simulink model "vf_ctrl"  (R2022a)
settings: Solver=FixedStepDiscrete  StartTime=0.0  StopTime=3  FixedStep=T_HF_TASK  RelTol=1e-3  EnableMultiTasking=on
PostLoadFcn:
  | run('init.m')
values from neighbouring files (symbols this model uses):
  INT16_MAX = 32767.0    [vf_ctrl_dd.sldd]
  INT16_MIN = -32768.0    [vf_ctrl_dd.sldd]
  MOTOR_F = 6.3E-6    [vf_ctrl_dd.sldd]
  MOTOR_J = 7.5E-6    [vf_ctrl_dd.sldd]
  MOTOR_PN = 2    [vf_ctrl_dd.sldd]
  MOTOR_PNF = 2.0    [vf_ctrl_dd.sldd]
  MOTOR_TL = 0.001    [vf_ctrl_dd.sldd]
  MOTOR_TYPE = 11.0    [vf_ctrl_dd.sldd]
  PWM_PERIOD_CYCLES = 7200.0    [vf_ctrl_dd.sldd]
  T_HF_TASK = 0.0001    [vf_ctrl_dd.sldd]
  VBUS = 24.0    [vf_ctrl_dd.sldd]
undefined symbols (not defined in the file or in its folder): DiscIntNeverNeededParam
libraries: mcbplantlib x1, autolibpmsmexterior x1
settings Model: DataDictionary=vf_ctrl_dd.sldd  Creator=lww186  LastModifiedBy=YJRQZ777
settings SolverCC: AutoInsertRateTranBlk=on
settings OptimizationCC: DefaultParameterBehavior=Inlined  EnhancedBackFolding=on  PassReuseOutputArgsAs=Individual arguments  ZeroExternalMemoryAtStartup=off  ZeroInternalMemoryAtStartup=off  OptimizeBlockOrder=speed  DifferentSizesBufferReuse=on  OptimizationCustomize=off  EfficientTunableParamExpr=on
settings DebuggingCC: ParameterTunabilityLossMsg=error  UnconnectedInputMsg=warning  UnconnectedOutputMsg=warning  UnconnectedLineMsg=warning
settings HardwareCC: ProdBitPerPointer=32  ProdBitPerSizeT=32  ProdBitPerPtrDiffT=32  ProdLargestAtomicInteger=Long  ProdLargestAtomicFloat=Double  ProdWordSize=32  ProdHWDeviceType=ARM Compatible->ARM Cortex-M
settings SFSimCC: MATLABDynamicMemAlloc=off
settings RTWCC: SystemTargetFile=ert.tlc  GenCodeOnly=on  TemplateMakefile=ert_default_tmf  GenerateReport=on  LaunchReport=on  DLArmComputeVersion=19.05
settings CodeAppCC: ForceParamTrailComments=on  IgnoreCustomStorageClasses=off  OperatorAnnotations=on  SimulinkDataObjDesc=on  SFDataObjDesc=on  InsertBlockDesc=on
settings ERTTargetCC: TargetLangStandard=C99 (ISO)  InlinedParameterPlacement=NonHierarchical  ERTCustomFileTemplate=example_file_process.tlc

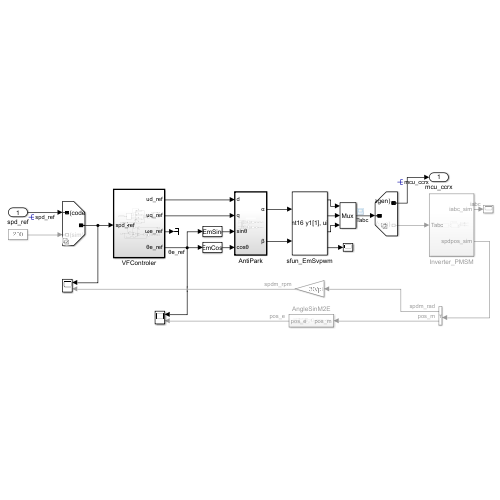
[thumbnail: Simulink's stored preview of the top-level diagram]
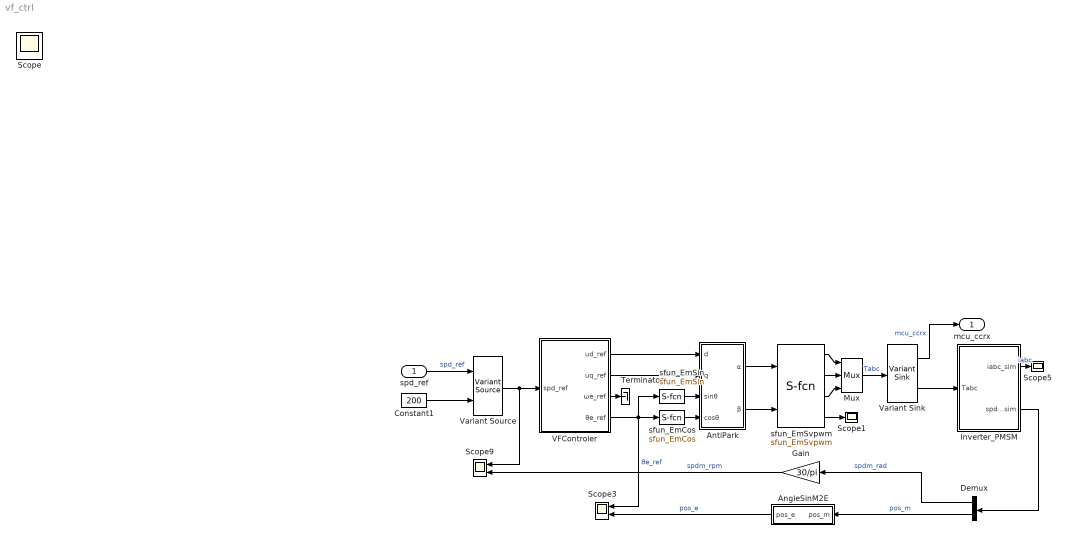
== system vf_ctrl ==
  spd_ref : Inport  OutDataTypeStr=int16
  AngleSinM2E : Subsystem
  AntiPark : Subsystem  TreatAsAtomicUnit=on
      settings: RTWFcnNameOpts=Use subsystem name  RTWFileNameOpts=Use subsystem name
  Constant1 : Constant  Value=200  OutDataTypeStr=int16
  Demux : Demux  Outputs=2
      settings: DisplayOption=none
  Gain : Gain  Gain=30/pi
  Inverter_PMSM : Subsystem
  Mux : Mux  Inputs=3
  Scope1 : Scope
  Scope3 : Scope  NumInputPorts=2
  Scope5 : Scope
  Scope9 : Scope  NumInputPorts=2
  Terminator : Terminator
  VFControler : Subsystem  TreatAsAtomicUnit=on  RTWFcnName=Vfcontroler  RTWFileName=Vfcontroler
      settings: RTWFcnNameOpts=Use subsystem name  RTWFileNameOpts=Use subsystem name
  Variant Sink : VariantSink  VariantControlMode=sim codegen switching  ShowConditionOnBlock=on
  Variant Source : VariantSource  VariantControlMode=sim codegen switching  ShowConditionOnBlock=on
  sfun_EmCos : S-Function  FunctionName=sfun_EmCos  SFunctionDeploymentMode=off  EnableBusSupport=off  mask(Legacy Function){SFunctionSpec=int16 y1 = EmCos( int16 u1 ), ShowSpec=on}
      mask prompts: ShowSpec "显示函数设定"
      mask help:
      | 此模块允许您调用由以下代码继承工具定义指定的已有函数:
      | def.SFunctionName = 'sfun_EmCos';
      | def.OutputFcnSpec = 'int16 y1 = EmCos( int16 u1 )';
      | def.HeaderFiles = {'em_sincos.h'};
      | def.SourceFiles = {'em_sincos.c'};
      | def.IncPaths = {'.\c_code'};
      mask Help: <p>此模块是由代码继承工具自动生成的。有关此工具的详细帮助，请调用<a href="matlab:legacy_code('help')"> legacy_code('help')</a>.</p>
      mask Callback ShowSpec:
      | if strcmp(get_param(gcbh, 'ShowSpec'), 'on')
      |   set_param(gcbh, 'MaskDisplay', sprintf('fprintf(''%s'');', get_param(gcbh, 'SFunctionSpec')));
      | else
      |   set_param(gcbh, 'MaskDisplay', sprintf('fprintf(''%s'');', get_param(gcbh, 'FunctionName')));
      | end
      mask Display: fprintf('int16 y1 = EmCos( int16 u1 )');
  sfun_EmSin : S-Function  FunctionName=sfun_EmSin  SFunctionDeploymentMode=off  EnableBusSupport=off  mask(Legacy Function){SFunctionSpec=int16 y1 = EmSin( int16 u1 ), ShowSpec=on}
      mask prompts: ShowSpec "显示函数设定"
      mask help:
      | 此模块允许您调用由以下代码继承工具定义指定的已有函数:
      | def.SFunctionName = 'sfun_EmSin';
      | def.OutputFcnSpec = 'int16 y1 = EmSin( int16 u1 )';
      | def.HeaderFiles = {'em_sincos.h'};
      | def.SourceFiles = {'em_sincos.c'};
      | def.IncPaths = {'.\c_code'};
      mask Help: <p>此模块是由代码继承工具自动生成的。有关此工具的详细帮助，请调用<a href="matlab:legacy_code('help')"> legacy_code('help')</a>.</p>
      mask Callback ShowSpec:
      | if strcmp(get_param(gcbh, 'ShowSpec'), 'on')
      |   set_param(gcbh, 'MaskDisplay', sprintf('fprintf(''%s'');', get_param(gcbh, 'SFunctionSpec')));
      | else
      |   set_param(gcbh, 'MaskDisplay', sprintf('fprintf(''%s'');', get_param(gcbh, 'FunctionName')));
      | end
      mask Display: fprintf('int16 y1 = EmSin( int16 u1 )');
  sfun_EmSvpwm : S-Function  FunctionName=sfun_EmSvpwm  SFunctionDeploymentMode=off  EnableBusSupport=off  mask(Legacy Function){SFunctionSpec=void EmSvpwm(int16 u1, int16 u2, uint16 y1[1], uint16 y2[1], uint16 y3[1], uint16 y4[1]), ShowSpec=on}
      mask prompts: ShowSpec "显示函数设定"
      mask help:
      | 此模块允许您调用由以下代码继承工具定义指定的已有函数:
      | def.SFunctionName = 'sfun_EmSvpwm';
      | def.OutputFcnSpec = 'void EmSvpwm(int16 u1, int16 u2, uint16 y1[1], uint16 y2[1], uint16 y3[1], uint16 y4[1])';
      | def.HeaderFiles = {'em_svpwm.h'};
      | def.SourceFiles = {'em_svpwm.c'};
      | def.IncPaths = {'..\code\MATLAB'};
      mask Help: <p>此模块是由代码继承工具自动生成的。有关此工具的详细帮助，请调用<a href="matlab:legacy_code('help')"> legacy_code('help')</a>.</p>
      mask Callback ShowSpec:
      | if strcmp(get_param(gcbh, 'ShowSpec'), 'on')
      |   set_param(gcbh, 'MaskDisplay', sprintf('fprintf(''%s'');', get_param(gcbh, 'SFunctionSpec')));
      | else
      |   set_param(gcbh, 'MaskDisplay', sprintf('fprintf(''%s'');', get_param(gcbh, 'FunctionName')));
      | end
      mask Display: fprintf('void EmSvpwm(int16 u1, int16 u2, uint16 y1[1], uint16 y2[1], uint16 y3[1], uint16 y4[1])');
  mcu_ccrx : Outport  OutDataTypeStr=uint16
  Scope : Scope
  wires:
  VFControler/2(uq_ref) -> AntiPark/2(q)
  Variant Sink/2 -> Inverter_PMSM/1(Tabc)
  sfun_EmSvpwm/3 -> Mux/3
  Demux/1 -> Gain/1  "spdm_rad"
  AngleSinM2E/1(pos_e) -> Scope3/2  "pos_e"
  Variant Source/1 -> VFControler/1(spd_ref), Scope9/1
  sfun_EmSvpwm/1 -> Mux/1
  Gain/1 -> Scope9/2  "spdm_rpm"
  sfun_EmCos/1 -> AntiPark/4(cosθ)
  Constant1/1 -> Variant Source/2
  AntiPark/1(α) -> sfun_EmSvpwm/1
  Variant Sink/1 -> mcu_ccrx/1  "mcu_ccrx"
  Demux/2 -> AngleSinM2E/1(pos_m)  "pos_m"
  Inverter_PMSM/1(iabc_sim) -> Scope5/1  "iabc"
  Inverter_PMSM/2(spdpos_sim) -> Demux/1
  sfun_EmSvpwm/4 -> Scope1/1
  Mux/1 -> Variant Sink/1  "Tabc"
  spd_ref/1 -> Variant Source/1  "spd_ref"
  sfun_EmSin/1 -> AntiPark/3(sinθ)
  AntiPark/2(β) -> sfun_EmSvpwm/2
  VFControler/1(ud_ref) -> AntiPark/1(d)
  sfun_EmSvpwm/2 -> Mux/2
  VFControler/4(θe_ref) -> sfun_EmCos/1, Scope3/1, sfun_EmSin/1  "θe_ref"
  VFControler/3(ωe_ref) -> Terminator/1

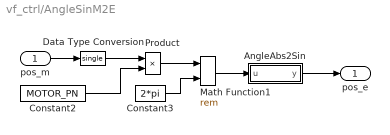
== system vf_ctrl/AngleSinM2E ==
  pos_m : Inport
  AngleAbs2Sin : MATLAB Function  TreatAsAtomicUnit=on
  Constant2 : Constant  Value=MOTOR_PN
  Constant3 : Constant  Value=2*pi  OutDataTypeStr=single
  Data Type Conversion : DataTypeConversion  OutDataTypeStr=single  SaturateOnIntegerOverflow=off  RndMeth=Floor
  Math Function1 : Math  Operator=rem
  Product : Product
  pos_e : Outport  OutDataTypeStr=single
  wires:
  Math Function1/1 -> AngleAbs2Sin/1(u)
  Product/1 -> Math Function1/1
  Constant3/1 -> Math Function1/2
  Constant2/1 -> Product/2
  pos_m/1 -> Data Type Conversion/1
  Data Type Conversion/1 -> Product/1
  AngleAbs2Sin/1(y) -> pos_e/1

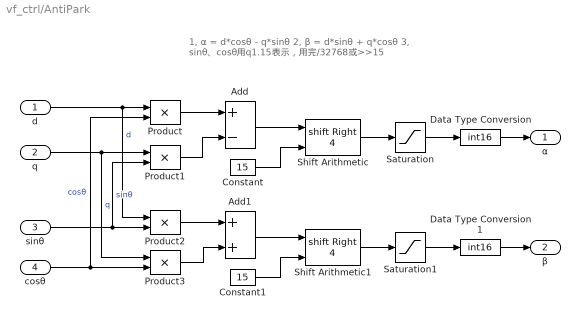
== system vf_ctrl/AntiPark ==
  note: 1, α = d*cosθ - q*sinθ
      | 2, β = d*sinθ + q*cosθ
      | 3, sinθ、cosθ用q1.15表示，用完/32768或>>15
  d : Inport  OutDataTypeStr=int16
  q : Inport  Port=2  OutDataTypeStr=int16
  sinθ : Inport  Port=3  OutDataTypeStr=int16
  cosθ : Inport  Port=4  OutDataTypeStr=int16
  Add : Sum  Inputs=+-
  Add1 : Sum
  Constant : Constant  Value=15  OutDataTypeStr=uint8
  Constant1 : Constant  Value=15  OutDataTypeStr=uint8
  Data Type Conversion : DataTypeConversion  OutDataTypeStr=int16  SaturateOnIntegerOverflow=off  RndMeth=Floor
  Data Type Conversion1 : DataTypeConversion  OutDataTypeStr=int16  SaturateOnIntegerOverflow=off  RndMeth=Floor
  Product{,1..3} (4 alike) : Product
  Saturation : Saturate  UpperLimit=INT16_MAX  LowerLimit=INT16_MIN
  Saturation1 : Saturate  UpperLimit=INT16_MAX  LowerLimit=INT16_MIN
  Shift Arithmetic : ArithShift  BitShiftNumberSource=Input port  BitShiftNumber=4  BitShiftDirection=Right
      settings: InputPortMap=u0,p1
  Shift Arithmetic1 : ArithShift  BitShiftNumberSource=Input port  BitShiftNumber=4  BitShiftDirection=Right
      settings: InputPortMap=u0,p1
  α : Outport  OutDataTypeStr=int16
  β : Outport  Port=2  OutDataTypeStr=int16
  wires:
  d/1 -> Product2/1, Product/1  "d"
  Add/1 -> Shift Arithmetic/1
  cosθ/1 -> Product/2, Product3/2  "cosθ"
  Constant/1 -> Shift Arithmetic/2
  Product1/1 -> Add/2
  q/1 -> Product3/1, Product1/1  "q"
  Product/1 -> Add/1
  sinθ/1 -> Product1/2, Product2/2  "sinθ"
  Add1/1 -> Shift Arithmetic1/1
  Data Type Conversion/1 -> α/1
  Constant1/1 -> Shift Arithmetic1/2
  Data Type Conversion1/1 -> β/1
  Product3/1 -> Add1/2
  Product2/1 -> Add1/1
  Shift Arithmetic/1 -> Saturation/1
  Saturation/1 -> Data Type Conversion/1
  Shift Arithmetic1/1 -> Saturation1/1
  Saturation1/1 -> Data Type Conversion1/1

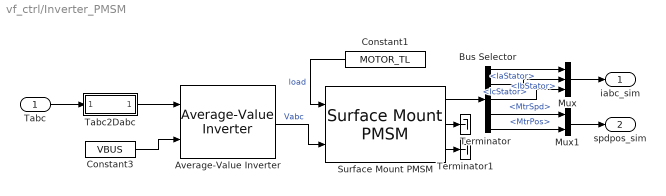
== system vf_ctrl/Inverter_PMSM ==
  Tabc : Inport
  Average-Value Inverter : mcbplantlib/Average-Value Inverter
  Bus Selector : BusSelector  OutputSignals=IaStator,IbStator,IcStator,MtrSpd,MtrPos
  Constant1 : Constant  Value=MOTOR_TL  OutDataTypeStr=single
  Constant3 : Constant  Value=VBUS  OutDataTypeStr=single
  Mux : Mux  Inputs=3
  Mux1 : Mux  Inputs=2
  Surface Mount PMSM : autolibpmsmexterior/Surface Mount PMSM  port_config=Torque  sim_type=Discrete  Ts=T_HF_TASK  P=MOTOR_PNF  Rs=MOTOR_RS  Ldq_=MOTOR_LS  KConstText=Back-emf constant (Ke):  lambda_pm=0.2205  Ke=MOTOR_KE  Kt=1.323  mechanical=[MOTOR_J, MOTOR_F, 0]  idq0=[0 0]  theta_init=0  omega_init=0  KConst=0.2205  lambda_pm_calc=0.016449  RefBlkName='autolibpmsmexterior/Surface Mount PMSM'  aMode=5  Ldq="[0.0017      0.0017]"
      settings: SourceProductBaseCode=PW,DR,MT,VE
  Tabc2Dabc : Subsystem
  Terminator : Terminator
  Terminator1 : Terminator
  iabc_sim : Outport
  spdpos_sim : Outport  Port=2
  wires:
  Tabc/1 -> Tabc2Dabc/1(Tabc)
  Tabc2Dabc/1(Dabc) -> Average-Value Inverter/1
  Constant3/1 -> Average-Value Inverter/2
  Average-Value Inverter/1 -> Surface Mount PMSM/2  "Vabc"
  Bus Selector/5 -> Mux1/2  "<MtrPos>"
  Constant1/1 -> Surface Mount PMSM/1  "load"
  Bus Selector/4 -> Mux1/1  "<MtrSpd>"
  Bus Selector/2 -> Mux/2  "<IbStator>"
  Bus Selector/3 -> Mux/3  "<IcStator>"
  Surface Mount PMSM/1 -> Bus Selector/1
  Mux/1 -> iabc_sim/1
  Bus Selector/1 -> Mux/1  "<IaStator>"
  Mux1/1 -> spdpos_sim/1
  Surface Mount PMSM/2 -> Terminator/1
  Surface Mount PMSM/3 -> Terminator1/1

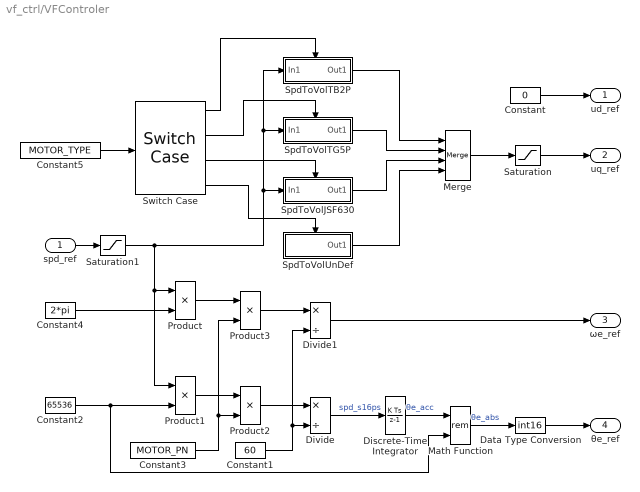
== system vf_ctrl/VFControler ==
  spd_ref : Inport  OutDataTypeStr=int16
  Constant : Constant  Value=0  OutDataTypeStr=int16
  Constant1 : Constant  Value=60  OutDataTypeStr=uint8
  Constant2 : Constant  Value=65536  OutDataTypeStr=int32
  Constant3 : Constant  Value=MOTOR_PN  OutDataTypeStr=uint8
  Constant4 : Constant  Value=2*pi  OutDataTypeStr=single
  Constant5 : Constant  Value=MOTOR_TYPE  OutDataTypeStr=uint8
  Data Type Conversion : DataTypeConversion  OutDataTypeStr=int16  SaturateOnIntegerOverflow=off  RndMeth=Floor
  Discrete-Time Integrator : DiscreteIntegrator  SampleTime=-1  OutDataTypeStr=int32  ICPrevOutput=DiscIntNeverNeededParam  ICPrevScaledInput=DiscIntNeverNeededParam
  Divide : Product  Inputs=*/  OutDataTypeStr=int32
  Divide1 : Product  Inputs=*/
  Math Function : Math  Operator=rem
  Merge : Merge  Inputs=4
  Product : Product
  Product1 : Product  OutDataTypeStr=int32
  Product2 : Product  OutDataTypeStr=int32
  Product3 : Product
  Saturation : Saturate  UpperLimit=INT16_MAX  LowerLimit=INT16_MIN
  Saturation1 : Saturate  UpperLimit=600  LowerLimit=-600
  SpdToVolJSF630 : Subsystem  TreatAsAtomicUnit=on
  SpdToVolTB2P : Subsystem  TreatAsAtomicUnit=on
  SpdToVolTG5P : Subsystem  TreatAsAtomicUnit=on
  SpdToVolUnDef : Subsystem  TreatAsAtomicUnit=on
  Switch Case : SwitchCase  CaseConditions={MOTOR_TYPE_TB2P,MOTOR_TYPE_TG5P60,MOTOR_TYPE_JSF630}
  ud_ref : Outport  OutDataTypeStr=int16
  uq_ref : Outport  Port=2  OutDataTypeStr=int16
  ωe_ref : Outport  Port=3  OutDataTypeStr=single
  θe_ref : Outport  Port=4  OutDataTypeStr=int16
  wires:
  Constant/1 -> ud_ref/1
  Merge/1 -> Saturation/1
  Saturation1/1 -> SpdToVolTB2P/1(In1), SpdToVolTG5P/1(In1), SpdToVolJSF630/1(In1), Product1/1, Product/1
  Saturation/1 -> uq_ref/1
  Constant2/1 -> Product1/2, Math Function/2
  Product1/1 -> Product2/1
  Constant3/1 -> Product2/2, Product3/2
  Product2/1 -> Divide/1
  Constant1/1 -> Divide1/2, Divide/2
  Divide/1 -> Discrete-Time Integrator/1  "spd_s16ps"
  Discrete-Time Integrator/1 -> Math Function/1  "θe_acc"
  Math Function/1 -> Data Type Conversion/1  "θe_abs"
  Data Type Conversion/1 -> θe_ref/1
  Constant4/1 -> Product/2
  Product3/1 -> Divide1/1
  Product/1 -> Product3/1
  Divide1/1 -> ωe_ref/1
  spd_ref/1 -> Saturation1/1
  Constant5/1 -> Switch Case/1
  SpdToVolTG5P/1(Out1) -> Merge/2
  SpdToVolTB2P/1(Out1) -> Merge/1
  SpdToVolUnDef/1(Out1) -> Merge/4
  SpdToVolJSF630/1(Out1) -> Merge/3
  Switch Case/1 -> SpdToVolTB2P/Action
  Switch Case/2 -> SpdToVolTG5P/Action
  Switch Case/3 -> SpdToVolJSF630/Action
  Switch Case/4 -> SpdToVolUnDef/Action

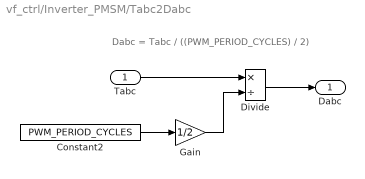
== system vf_ctrl/Inverter_PMSM/Tabc2Dabc ==
  note: Dabc = Tabc / ((PWM_PERIOD_CYCLES) / 2)
  Tabc : Inport  OutDataTypeStr=uint16
  Constant2 : Constant  Value=PWM_PERIOD_CYCLES  OutDataTypeStr=single
  Divide : Product  Inputs=*/
  Gain : Gain  Gain=1/2
  Dabc : Outport  OutDataTypeStr=single
  wires:
  Tabc/1 -> Divide/1
  Divide/1 -> Dabc/1
  Constant2/1 -> Gain/1
  Gain/1 -> Divide/2

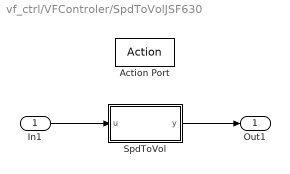
== system vf_ctrl/VFControler/SpdToVolJSF630 ==
  In1 : Inport
  Action Port : ActionPort  ActionPortLabel=case [ 21 ]:
  SpdToVol : MATLAB Function  TreatAsAtomicUnit=on
  Out1 : Outport
  wires:
  In1/1 -> SpdToVol/1(u)
  SpdToVol/1(y) -> Out1/1

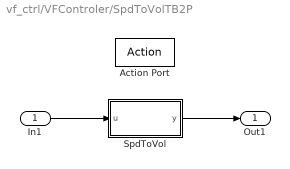
== system vf_ctrl/VFControler/SpdToVolTB2P ==
  In1 : Inport
  Action Port : ActionPort  ActionPortLabel=case [ 11 ]:
  SpdToVol : MATLAB Function  TreatAsAtomicUnit=on
  Out1 : Outport
  wires:
  In1/1 -> SpdToVol/1(u)
  SpdToVol/1(y) -> Out1/1

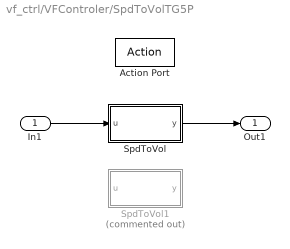
== system vf_ctrl/VFControler/SpdToVolTG5P ==
  In1 : Inport
  Action Port : ActionPort  ActionPortLabel=case [ 3 ]:
  SpdToVol : MATLAB Function  TreatAsAtomicUnit=on
  SpdToVol1 : MATLAB Function  Commented=on  TreatAsAtomicUnit=on
  Out1 : Outport
  wires:
  In1/1 -> SpdToVol/1(u)
  SpdToVol/1(y) -> Out1/1

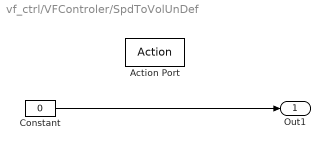
== system vf_ctrl/VFControler/SpdToVolUnDef ==
  Action Port : ActionPort  ActionPortLabel=default:
  Constant : Constant  Value=0  OutDataTypeStr=int16
  Out1 : Outport
  wires:
  Constant/1 -> Out1/1

== matlab function vf_ctrl/VFControler/SpdToVolTB2P/SpdToVol ==
  data: u input int16; y output int16
function y = fcn(u)
% s16:
u_abs = u;
if(u_abs < 0)
    u_abs = -u_abs;
end

if(u_abs == 0)
    y = int16(0);
elseif(u_abs <= 100)
    y = int16(2955);
elseif(u_abs <= 200)
    y = int16(3547);
elseif(u_abs <= 300)
    y = int16(4138);
elseif(u_abs <= 400)
    y = int16(4729);
elseif(u_abs <= 500)
    y = int16(5320);
elseif(u_abs <= 550)
    y = int16(5911);
elseif(u_abs <= 600)
    y = int16(6503);
else    
    y = int16(6503);
end

if(u < 0)
    y = -y;
end

== matlab function vf_ctrl/AngleSinM2E/AngleAbs2Sin ==
  data: u input; y output
function y = fcn(u)
if (u > pi)
    y = u - 2*pi;
elseif (u < -pi)
    y = u + 2*pi;
else
    y = u;
end

== matlab function vf_ctrl/VFControler/SpdToVolTG5P/SpdToVol ==
  data: u input int16; y output int16
function y = fcn(u)
% s16:
u_abs = u;
if(u_abs < 0)
    u_abs = -u_abs;
end

if(u_abs == 0)
    y = int16(0);
elseif(u_abs <= 200)
    y = int16(3700);
elseif(u_abs <= 300)
    y = int16(4300);
elseif(u_abs <= 350)
    y = int16(4900);
elseif(u_abs <= 450)
    y = int16(5500);
elseif(u_abs <= 600)
    y = int16(6503);
else    
    y = int16(6503);
end

if(u < 0)
    y = -y;
end

== matlab function vf_ctrl/VFControler/SpdToVolTG5P/SpdToVol1 ==
  data: u input int16; y output int16
function y = fcn(u)
% s16:
u_abs = u;
if(u_abs < 0)
    u_abs = -u_abs;
end

if(u_abs == 0)
    y = int16(0);
elseif(u_abs <= 150)
    y = int16(2955);
elseif(u_abs <= 250)
    y = int16(3547);
elseif(u_abs <= 300)
    y = int16(4138);
elseif(u_abs <= 400)
    y = int16(4729);
elseif(u_abs <= 500)
    y = int16(5320);
elseif(u_abs <= 550)
    y = int16(5911);
elseif(u_abs <= 600)
    y = int16(6503);
else    
    y = int16(6503);
end

if(u < 0)
    y = -y;
end

== matlab function vf_ctrl/VFControler/SpdToVolJSF630/SpdToVol ==
  data: u input int16; y output int16
function y = fcn(u)
% s16:
u_abs = u;
if(u_abs < 0)
    u_abs = -u_abs;
end

if(u_abs == 0)
    y = int16(0);
elseif(u_abs <= 100)
    y = int16(3277);
elseif(u_abs <= 300)
    y = int16(4916);
elseif(u_abs <= 400)
    y = int16(5911);
elseif(u_abs <= 500)
    y = int16(6503);
elseif(u_abs <= 600)
    y = int16(7500);
else    
    y = int16(7500);
end

if(u < 0)
    y = -y;
end
